simulink library "csc_sensors_mtv_lib"  (R2014b)
settings: Solver=ode45  SolverMode=SingleTasking  StartTime=0.0  StopTime=10.0  RelTol=1e-3
undefined symbols (not defined in the file or in its folder): cam_cam1_lander_dcm, cam_cam1_lander_quat, cam_cam1_pos_in_lander, cam_processing_delay_cycles
libraries: util_common_lib x3, util_info_lib x1, csc_cam_camera_system_lib x1, csc_gps_piksi_model_lib x1, csc_ldr_flir_lidar_lib x1, csc_mem_cab_integrated_mems_lib x1, csc_sei_sensonor_external_imu_lib x1, csc_sta_star_tracker_lib x1
settings Model: ExtModeAutoUpdateStatusClock=off  Creator=hcannon  LastModifiedBy=mstewart

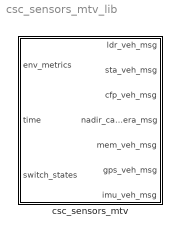
== system csc_sensors_mtv_lib ==
  csc_sensors_mtv : Subsystem

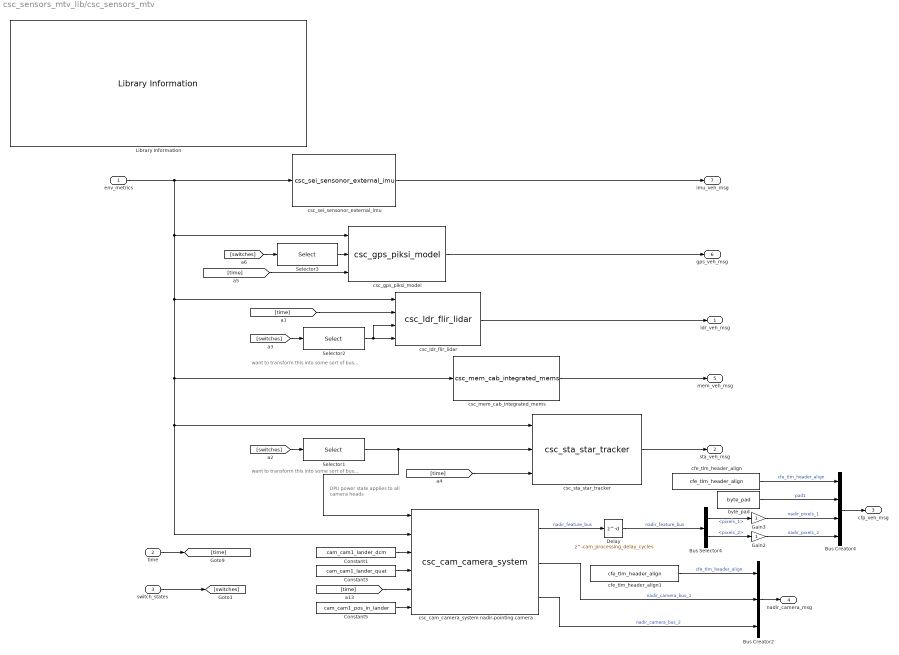
== system csc_sensors_mtv_lib/csc_sensors_mtv ==
  note: want to transform this into some sort of bus...
  note: want to transform this into some sort of bus...
  note: DPU power state applies
      | to all camera heads
  env_metrics : Inport
  time : Inport  Port=2
  switch_states : Inport  Port=3
  Bus Creator2 : BusCreator  Inputs=3  NonVirtualBus=on
  Bus Creator4 : BusCreator  OutDataTypeStr=Bus: cfp_veh_msg  NonVirtualBus=on
  Bus Selector4 : BusSelector  OutputSignals=pixels_1,pixels_2
  Constant1 : Constant  Value=cam_cam1_lander_dcm
  Constant3 : Constant  Value=cam_cam1_lander_quat
  Constant5 : Constant  Value=cam_cam1_pos_in_lander
  Delay : Delay  DelayLength=cam_processing_delay_cycles
  Gain2 : Gain
  Gain3 : Gain
  Library Information : util_info_lib/Library Information  owner='NONE'
  Selector1 : Selector  InputPortWidth=swm_num_switches
  Selector2 : Selector  InputPortWidth=swm_num_switches  Indices=2
  Selector3 : Selector  InputPortWidth=swm_num_switches  Indices=2
  byte_pad : util_common_lib/byte_pad  n_bytes=4
  cfe_tlm_header_align : util_common_lib/cfe_tlm_header_align
  cfe_tlm_header_align1 : util_common_lib/cfe_tlm_header_align
  csc_cam_camera_system nadir-pointing camera : csc_cam_camera_system_lib/csc_cam_camera_system
  csc_gps_piksi_model : csc_gps_piksi_model_lib/csc_gps_piksi_model
  csc_ldr_flir_lidar : csc_ldr_flir_lidar_lib/csc_ldr_flir_lidar
  csc_mem_cab_integrated_mems : csc_mem_cab_integrated_mems_lib/csc_mem_cab_integrated_mems
  csc_sei_sensonor_external_imu : csc_sei_sensonor_external_imu_lib/csc_sei_sensonor_external_imu
  csc_sta_star_tracker : csc_sta_star_tracker_lib/csc_sta_star_tracker
  ldr_veh_msg : Outport
  sta_veh_msg : Outport  Port=2
  cfp_veh_msg : Outport  Port=3
  nadir_camera_msg : Outport  Port=4
  mem_veh_msg : Outport  Port=5
  gps_veh_msg : Outport  Port=6
  imu_veh_msg : Outport  Port=7
  wires:
  csc_sei_sensonor_external_imu/1 -> imu_veh_msg/1
  csc_gps_piksi_model/1 -> gps_veh_msg/1
  Selector3/1 -> csc_gps_piksi_model/2
  [switches] -> Selector3/1
  [time] -> csc_gps_piksi_model/3
  csc_mem_cab_integrated_mems/1 -> mem_veh_msg/1
  [time] -> csc_sta_star_tracker/3
  Selector2/1 -> csc_ldr_flir_lidar/4, csc_ldr_flir_lidar/3
  [switches] -> Selector2/1
  [switches] -> Selector1/1
  switch_states/1 -> [switches]
  Selector1/1 -> csc_cam_camera_system nadir-pointing camera/1, csc_sta_star_tracker/2
  csc_cam_camera_system nadir-pointing camera/3 -> Bus Creator2/3  "nadir_camera_bus_2"
  cfe_tlm_header_align1/1 -> Bus Creator2/1  "cfe_tlm_header_align"
  cfe_tlm_header_align/1 -> Bus Creator4/1  "cfe_tlm_header_align"
  byte_pad/1 -> Bus Creator4/2  "pad1"
  Bus Selector4/2 -> Gain2/1  "<pixels_2>"
  Constant5/1 -> csc_cam_camera_system nadir-pointing camera/6
  [time] -> csc_ldr_flir_lidar/2
  [time] -> csc_cam_camera_system nadir-pointing camera/5
  time/1 -> [time]
  Constant3/1 -> csc_cam_camera_system nadir-pointing camera/4
  Bus Creator2/1 -> nadir_camera_msg/1
  csc_ldr_flir_lidar/1 -> ldr_veh_msg/1
  csc_sta_star_tracker/1 -> sta_veh_msg/1
  env_metrics/1 -> csc_gps_piksi_model/1, csc_cam_camera_system nadir-pointing camera/2, csc_sta_star_tracker/1, csc_mem_cab_integrated_mems/1, csc_ldr_flir_lidar/1, csc_sei_sensonor_external_imu/1
  Constant1/1 -> csc_cam_camera_system nadir-pointing camera/3
  csc_cam_camera_system nadir-pointing camera/1 -> Delay/1  "nadir_feature_bus"
  csc_cam_camera_system nadir-pointing camera/2 -> Bus Creator2/2  "nadir_camera_bus_1"
  Bus Creator4/1 -> cfp_veh_msg/1
  Delay/1 -> Bus Selector4/1  "nadir_feature_bus"
  Bus Selector4/1 -> Gain3/1  "<pixels_1>"
  Gain3/1 -> Bus Creator4/3  "nadir_pixels_1"
  Gain2/1 -> Bus Creator4/4  "nadir_pixels_2"
